simulink model "ROPOD_4Wheel_TdistZMPC_cntr_EC"  (R2017b)
settings: Solver=ode1  StartTime=0.0  StopTime=Tfinal  FixedStep=Ts  RelTol=1e-3  EnableMultiTasking=on
PreLoadFcn:
  | init_model
InitFcn:
  | init_model
values from neighbouring files (symbols this model uses):
  b_cx = 70.26    [RoPod_parameters.mat]
  b_cy = 36.5    [RoPod_parameters.mat]
  FFtheta_intia = 0    [init_model.m]
  FFxy_mass = 80    [init_model.m]
  I_fhz_dtheta_cntr = 0.5    [init_model.m]
  I_fhz_dvarphi_cntr = 0    [init_model.m]
  I_fhz_dxdy_cntr = 0.25    [init_model.m]
  k_cx = 4300    [RoPod_parameters.mat]
  k_cy = 4489    [RoPod_parameters.mat]
  K_gain_dtheta_cntr = 150    [init_model.m]
  K_gain_dvarphi_cntr = 0.05    [init_model.m]
  K_gain_dxdy_cntr = 200    [init_model.m]
  LL_wp_fhz_dtheta_cntr = 20    [init_model.m]
  LL_wp_fhz_dvarphi_cntr = 20    [init_model.m]
  LL_wp_fhz_dxdy_cntr = 20    [init_model.m]
  LL_wz_fhz_dtheta_cntr = 20    [init_model.m]
  LL_wz_fhz_dvarphi_cntr = 2    [init_model.m]
  LL_wz_fhz_dxdy_cntr = 20    [init_model.m]
  LPF_fhz_dtheta_cntr = 100    [init_model.m]
  LPF_fhz_dvarphi_cntr = 100    [init_model.m]
  LPF_fhz_dxdy_cntr = 100    [init_model.m]
  max_hw_tau = 7.0    (= 7)    [init_model.m]
  max_ropod_acc_theta = 1.6    [init_model.m]
  max_ropod_acc_xy = 1.0    (= 1)    [init_model.m]
  max_ropod_vel_theta = 1.6    [init_model.m]
  max_ropod_vel_xy = 1.0    (= 1)    [init_model.m]
  max_sw_current = 10    [init_model.m]
  Nwheels = 4    [init_model.m]
  pivot_offs_sws = [2.21 1.873 2.001 3.508]    [init_model.m]
  SW_COM1_ENABLE1 = hex2dec('0001')    [init_model.m]
  SW_COM1_ENABLE2 = hex2dec('0002')    [init_model.m]
  SW_COM1_MODE_TORQUE = bitshift(hex2dec('0000'),2)    [init_model.m]
  SW_COM1_MODE_VELOCITY = bitshift(hex2dec('0002'),2)    [init_model.m]
  SW_COM1_USE_TS = hex2dec('8000')    [init_model.m]
  sw_tau_2_curr = 1/motor_physical_parameters.torqueconstant.value    [init_model.m]
  Taucompfactor = 2.0    (= 2)    [init_model.m]
  Tinit = 1*Tslot    [init_model.m]
  Ts = 0.001    [init_model.m]
  Ts_MPC = 0.001    [init_model.m]
  xA = [1 -1 0 0 0 0 0.0206696424966 -0.0206696424966 0 0 0.0298227588181 -0.0298227588181 ... (4080 elements, 102x40)]    [ZMPCx_parameters.mat]
  xBd_dis = [1.12932348493e-06 0.000225071897401 0 0]    [ZMPCx_parameters.mat]
  xF = [0 0 0 0 0 0 0 0 0 0 0 0 ... (80 elements, 20x4)]    [ZMPCx_parameters.mat]
  xH = [20 0 0 0 0 0 0 0 0 0 0 0 ... (1600 elements, 40x40)]    [ZMPCx_parameters.mat]
  xPhi = [0.995143909015 -0.967809158823 0 0 0.980727027327 -1.91066813489 0 0 0.957042868744 -2.81984596436 0 0 ... (320 elements, 80x4)]    [ZMPCx_parameters.mat]
  xrho = 144000    [ZMPCx_parameters.mat]
  xW = [0 0 -4300 4300 0 0 -4211.12053726 4211.12053726 0 0 -4082.88267435 4082.88267435 ... (328 elements, 82x4)]    [ZMPCx_parameters.mat]
  yA = [1 -1 0 0 0 0 0.0146537039222 -0.0146537039222 0 0 0.0255124036215 -0.0255124036215 ... (4080 elements, 102x40)]    [ZMPCy_parameters.mat]
  yBd_dis = [1.24492522358e-06 0.000248362591603 0 0]    [ZMPCy_parameters.mat]
  yF = [0.00191047141222 0.00156448969707 0.00119761396088 0.000813779538874 0.00041715000072 1.20724055612e-05 -0.00039696993291 -0.000805406662726 -0.00120863105559 -0.00160205155743 -0.00198114365531 -0.00234150147928 ... (80 elements, 20x4)]    [ZMPCy_parameters.mat]
  yH = [2.00000002801 0 2.31602594113e-08 0 1.80085634996e-08 0 1.26053094289e-08 0 7.00898668547e-09 0 1.2808124932e-09 0 ... (1600 elements, 40x40)]    [ZMPCy_parameters.mat]
  yPhi = [0.994411530671 -1.11489967371 0 0 0.977778317439 -2.20691845877 0 0 0.950389393786 -3.2640842851 0 0 ... (320 elements, 80x4)]    [ZMPCy_parameters.mat]
  yrho = 10000    [ZMPCy_parameters.mat]
  yW = [0 0 -4489 4489 0 0 -4423.21952309 4423.21952309 0 0 -4308.69434324 4308.69434324 ... (328 elements, 82x4)]    [ZMPCy_parameters.mat]
undefined symbols (not defined in the file or in its folder): DiscIntNeverNeededParam, Fd_max, Fd_min, Fr_max, Fr_min, ropod_kinmodel_param
libraries: cstblocks x85, simulink x41, SOEM_EtherCAT_Lib x5
(part 1 of 5)
settings Model: SimulationMode=external  Creator=cesar  LastModifiedBy=root
settings OptimizationCC: PassReuseOutputArgsThreshold=0  MaxStackSize=64
settings DebuggingCC: ParameterTunabilityLossMsg=error
settings HardwareCC: ProdBitPerLong=64  ProdHWDeviceType=Intel->x86-64 (Linux 64)  TargetBitPerLong=64  TargetBitPerPointer=64  TargetBitPerSizeT=64  TargetBitPerPtrDiffT=64  TargetLargestAtomicFloat=Float  TargetIntDivRoundTo=Zero  TargetEndianess=LittleEndian  TargetWordSize=64  TargetHWDeviceType=Intel->x86-64 (Linux 64)
settings SFSimCC: MATLABDynamicMemAlloc=off
settings RTWCC: SystemTargetFile=mttarget.tlc  MakeCommand="make_rtw  CC=\"ccache gcc\" OPTS=\"-DNETIF_ID=0 -DTEST_CONN_MODEL -D_GNU_SOURCE -DPRIO=99\""  TemplateMakefile=mt_unix.tmf  Description=Generic Real-Time Target  CustomInclude=/usr/local/include/soem  Toolchain=Catkin  BuildConfiguration=Faster Runs  RTWCompilerOptimization=Custom  RTWCustomCompilerOptimizations=-O2 -g -W
settings RTWCC: CustomLibrary=|
  | /usr/local/lib/libsoem.so
  | libgamepad.so.1
settings CodeAppCC: ForceParamTrailComments=on  OperatorAnnotations=on
settings GRTTargetCC: TargetLangStandard=C89/C90 (ANSI)  UseToolchainInfoCompliant=off  ExtMode=on

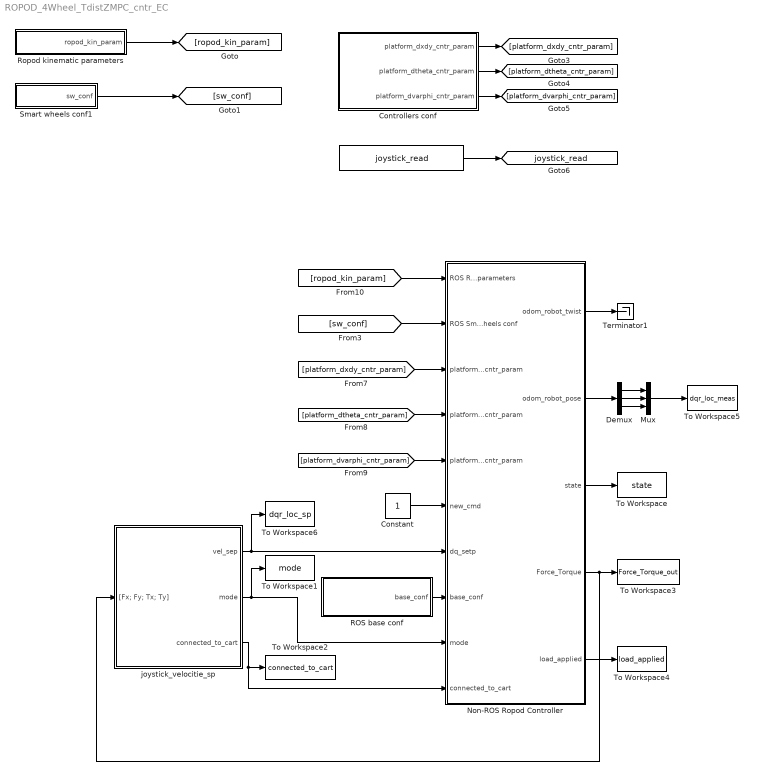
== system ROPOD_4Wheel_TdistZMPC_cntr_EC ==
  " " : S-Function  FunctionName=joystick_read  SFunctionDeploymentMode=off  EnableBusSupport=off  mask(Legacy Function){SFunctionSpec=double y1 = read_joystick(), ShowSpec=off}
      mask prompts: ShowSpec "Display function specification"
      mask help:
      | This block allows you to call the legacy functions specified by the following Legacy Code Tool definition:
      | def.SFunctionName = 'joystick_read';
      | def.OutputFcnSpec = 'double y1 = read_joystick()';
      | def.StartFcnSpec = 'void init()';
      | def.HeaderFiles = {'joystick.h', 'stdio.h', 'ncurses.h', 'gamepad.h'};
      | def.SourceFiles = {'joystick.c'};
      | def.HostLibFiles = {'libgamepad.so.1'};
      mask Help: <p>This block was generated automatically by the Legacy Code Tool. For detailed help on this tool, call<a href="matlab:legacy_code('help')"> legacy_code('help')</a>.</p>
      mask Callback ShowSpec:
      | if strcmp(get_param(gcbh, 'ShowSpec'), 'on')
      |   set_param(gcbh, 'MaskDisplay', sprintf('fprintf(''%s'');', get_param(gcbh, 'SFunctionSpec')));
      | else
      |   set_param(gcbh, 'MaskDisplay', sprintf('fprintf(''%s'');', get_param(gcbh, 'FunctionName')));
      | end
      mask Display: fprintf('joystick_read');
  Constant : Constant
  Controllers conf : Subsystem
  Demux : Demux  Outputs=3
  Mux : Mux  Inputs=3
  Non-ROS Ropod Controller : Subsystem
  ROS base conf : Subsystem
  Ropod kinematic parameters : Subsystem
  Smart wheels conf1 : Subsystem
  Terminator1 : Terminator
  To Workspace : ToWorkspace  VariableName=state  SampleTime=-1
      settings: Save2DSignal=2-D array (concatenate along first dimension)
  To Workspace1 : ToWorkspace  VariableName=mode  SampleTime=-1
      settings: Save2DSignal=2-D array (concatenate along first dimension)
  To Workspace2 : ToWorkspace  VariableName=connected_to_cart  SampleTime=-1
      settings: Save2DSignal=2-D array (concatenate along first dimension)
  To Workspace3 : ToWorkspace  VariableName=Force_Torque_out  SampleTime=-1
      settings: Save2DSignal=2-D array (concatenate along first dimension)
  To Workspace4 : ToWorkspace  VariableName=load_applied  SampleTime=-1
      settings: Save2DSignal=2-D array (concatenate along first dimension)
  To Workspace5 : ToWorkspace  VariableName=dqr_loc_meas  SampleTime=-1
      settings: Save2DSignal=2-D array (concatenate along first dimension)
  To Workspace6 : ToWorkspace  VariableName=dqr_loc_sp  SampleTime=-1
      settings: Save2DSignal=2-D array (concatenate along first dimension)
  joystick_velocitie_sp : Subsystem
  tag scope: joystick_read=global
  wires:
  Mux/1 -> To Workspace5/1
  Constant/1 -> Non-ROS Ropod Controller/6(new_cmd)
  " "/1 -> [joystick_read]
  [platform_dtheta_cntr_param] -> Non-ROS Ropod Controller/4(platform_dtheta_cntr_param)
  Non-ROS Ropod Controller/2(odom_robot_pose) -> Demux/1
  Demux/2 -> Mux/2
  [platform_dxdy_cntr_param] -> Non-ROS Ropod Controller/3(platform_dxdy_cntr_param)
  [platform_dvarphi_cntr_param] -> Non-ROS Ropod Controller/5(platform_dvarphi_cntr_param)
  Controllers conf/3(platform_dvarphi_cntr_param) -> [platform_dvarphi_cntr_param]
  Demux/3 -> Mux/3
  [ropod_kin_param] -> Non-ROS Ropod Controller/1(ROS Ropod kinematic parameters)
  Controllers conf/1(platform_dxdy_cntr_param) -> [platform_dxdy_cntr_param]
  Controllers conf/2(platform_dtheta_cntr_param) -> [platform_dtheta_cntr_param]
  [sw_conf] -> Non-ROS Ropod Controller/2(ROS Smart wheels conf)
  Ropod kinematic parameters/1(ropod_kin_param) -> [ropod_kin_param]
  Smart wheels conf1/1(sw_conf) -> [sw_conf]
  Non-ROS Ropod Controller/1(odom_robot_twist) -> Terminator1/1
  Demux/1 -> Mux/1
  ROS base conf/1(base_conf) -> Non-ROS Ropod Controller/8(base_conf)
  joystick_velocitie_sp/1(vel_sep) -> Non-ROS Ropod Controller/7(dq_setp), To Workspace6/1
  joystick_velocitie_sp/2(mode) -> Non-ROS Ropod Controller/9(mode), To Workspace1/1
  joystick_velocitie_sp/3(connected_to_cart) -> To Workspace2/1, Non-ROS Ropod Controller/10(connected_to_cart)
  Non-ROS Ropod Controller/3(state) -> To Workspace/1
  Non-ROS Ropod Controller/4(Force_Torque) -> joystick_velocitie_sp/1("[Fx; Fy; Tx; Ty]"), To Workspace3/1
  Non-ROS Ropod Controller/5(load_applied) -> To Workspace4/1

== system ROPOD_4Wheel_TdistZMPC_cntr_EC/Controllers conf ==
  Bus Creator : BusCreator  Inputs=5
  Bus Creator1 : BusCreator  Inputs=5
  Bus Creator2 : BusCreator  Inputs=5
  Constant1 : Constant  Value=I_fhz_dxdy_cntr
  Constant10 : Constant  Value=K_gain_dtheta_cntr
  Constant11 : Constant  Value=K_gain_dvarphi_cntr
  Constant12 : Constant  Value=I_fhz_dvarphi_cntr
  Constant13 : Constant  Value=LL_wp_fhz_dvarphi_cntr
  Constant14 : Constant  Value=LL_wz_fhz_dvarphi_cntr
  Constant15 : Constant  Value=LPF_fhz_dvarphi_cntr
  Constant2 : Constant  Value=LL_wp_fhz_dxdy_cntr
  Constant3 : Constant  Value=LL_wz_fhz_dxdy_cntr
  Constant4 : Constant  Value=LPF_fhz_dxdy_cntr
  Constant5 : Constant  Value=I_fhz_dtheta_cntr
  Constant6 : Constant  Value=LL_wp_fhz_dtheta_cntr
  Constant7 : Constant  Value=K_gain_dxdy_cntr
  Constant8 : Constant  Value=LL_wz_fhz_dtheta_cntr
  Constant9 : Constant  Value=LPF_fhz_dtheta_cntr
  platform_dxdy_cntr_param : Outport
  platform_dtheta_cntr_param : Outport  Port=2
  platform_dvarphi_cntr_param : Outport  Port=3
  wires:
  Constant2/1 -> Bus Creator/4  "LL_pole_fhz"
  Constant4/1 -> Bus Creator/5  "LPF_fhz"
  Bus Creator/1 -> platform_dxdy_cntr_param/1
  Constant1/1 -> Bus Creator/2  "I_freq_hz"
  Constant3/1 -> Bus Creator/3  "LL_zero_fhz"
  Constant7/1 -> Bus Creator/1  "P_gain"
  Bus Creator1/1 -> platform_dtheta_cntr_param/1
  Bus Creator2/1 -> platform_dvarphi_cntr_param/1
  Constant5/1 -> Bus Creator1/2  "I_freq_hz"
  Constant6/1 -> Bus Creator1/4  "LL_pole_fhz"
  Constant10/1 -> Bus Creator1/1  "P_gain"
  Constant8/1 -> Bus Creator1/3  "LL_zero_fhz"
  Constant9/1 -> Bus Creator1/5  "LPF_fhz"
  Constant15/1 -> Bus Creator2/5  "LPF_fhz"
  Constant12/1 -> Bus Creator2/2  "I_freq_hz"
  Constant14/1 -> Bus Creator2/3  "LL_zero_fhz"
  Constant11/1 -> Bus Creator2/1  "P_gain"
  Constant13/1 -> Bus Creator2/4  "LL_pole_fhz"

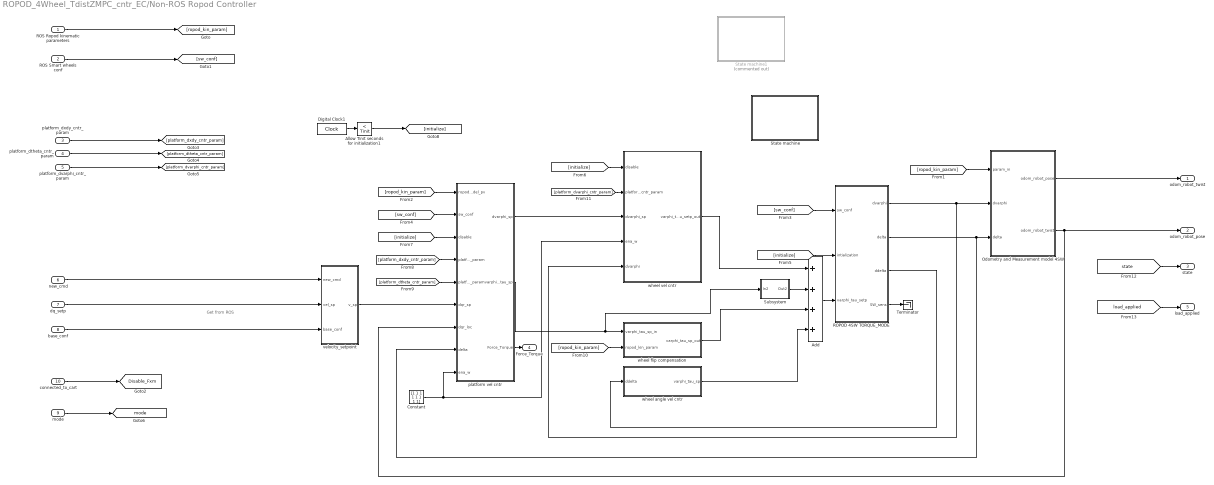
== system ROPOD_4Wheel_TdistZMPC_cntr_EC/Non-ROS Ropod Controller ==
  note: Get from ROS
  ROS Ropod kinematic parameters : Inport
  ROS Smart wheels conf : Inport  Port=2
  platform_dxdy_cntr_param : Inport  Port=3
  platform_dtheta_cntr_param : Inport  Port=4
  platform_dvarphi_cntr_param : Inport  Port=5
  new_cmd : Inport  Port=6
  dq_setp : Inport  Port=7
  base_conf : Inport  Port=8
  mode : Inport  Port=9
  connected_to_cart : Inport  Port=10
  Add : Sum  Inputs=++++
  Allow Tinit seconds for initialization1 : simulink/Logic and Bit Operations/Compare To Constant  relop=<  const=Tinit  OutDataTypeStr=boolean
  Constant : Constant  Value=[1 1 1 1 1 1 1 1]
  Digital Clock1 : DigitalClock  SampleTime=Ts
  Odometry and Measurement model 4SW : Subsystem
  ROPOD 4SW TORQUE_MODE : Subsystem
  State machine : Subsystem
  State machine1 : Subsystem  Commented=on
  Subsystem : Subsystem
  Terminator : Terminator
  platform vel cntr : Subsystem
  velocity_setpoint : Subsystem
  wheel angle vel cntr : Subsystem
  wheel flip compensation : Subsystem
  wheel vel cntr : Subsystem
  odom_robot_twist : Outport
  odom_robot_pose : Outport  Port=2
  state : Outport  Port=3
  Force_Torque : Outport  Port=4
  load_applied : Outport  Port=5
  tag scope: Disable_Fxm=global, mode=global
  wires:
  [sw_conf] -> ROPOD 4SW TORQUE_MODE/1(sw_conf)
  ROPOD 4SW TORQUE_MODE/3(ddelta) -> wheel angle vel cntr/1(ddelta)
  [initialize] -> wheel vel cntr/1(disable)
  base_conf/1 -> velocity_setpoint/3(base_conf)
  Digital Clock1/1 -> Allow Tinit seconds for initialization1/1
  [sw_conf] -> platform vel cntr/2(sw_conf)
  [platform_dvarphi_cntr_param] -> wheel vel cntr/2(platform_dxdy_cntr_param)
  wheel angle vel cntr/1(varphi_tau_sp) -> Add/4
  ROPOD 4SW TORQUE_MODE/2(delta) -> Odometry and Measurement model 4SW/3(delta), platform vel cntr/8(delta)
  [platform_dtheta_cntr_param] -> platform vel cntr/5(platform_dtheta_cntr_param)
  platform vel cntr/2(varphi_tau_sp) -> Subsystem/1(In2), wheel flip compensation/1(varphi_tau_sp_in)
  Add/1 -> ROPOD 4SW TORQUE_MODE/3(varphi_tau_setp)
  [platform_dxdy_cntr_param] -> platform vel cntr/4(platform_dxdy_cntr_param)
  [ropod_kin_param] -> platform vel cntr/1(ropod_kinmodel_pv)
  velocity_setpoint/1(v_sp) -> platform vel cntr/6(dqr_sp)
  wheel flip compensation/1(varphi_tau_sp_out) -> Add/3
  ROS Smart wheels conf/1 -> [sw_conf]
  platform_dvarphi_cntr_param/1 -> [platform_dvarphi_cntr_param]
  Odometry and Measurement model 4SW/1(odom_robot_pose) -> odom_robot_twist/1
  [ropod_kin_param] -> Odometry and Measurement model 4SW/1(param_in)
  [initialize] -> platform vel cntr/3(disable)
  ROPOD 4SW TORQUE_MODE/4(SW_sens) -> Terminator/1
  platform_dxdy_cntr_param/1 -> [platform_dxdy_cntr_param]
  ROS Ropod kinematic parameters/1 -> [ropod_kin_param]
  [initialize] -> ROPOD 4SW TORQUE_MODE/2(intialization)
  [ropod_kin_param] -> wheel flip compensation/2(ropod_kin_param)
  platform vel cntr/1(dvarphi_sp) -> wheel vel cntr/3(dvarphi_sp)
  Odometry and Measurement model 4SW/2(odom_robot_twist) -> odom_robot_pose/1, platform vel cntr/7(dqr_loc)
  ROPOD 4SW TORQUE_MODE/1(dvarphi) -> Odometry and Measurement model 4SW/2(dvarphi), wheel vel cntr/5(dvarphi)
  platform_dtheta_cntr_param/1 -> [platform_dtheta_cntr_param]
  new_cmd/1 -> velocity_setpoint/1(new_cmd)
  dq_setp/1 -> velocity_setpoint/2(vel_sp)
  Constant/1 -> wheel vel cntr/4(ena_w), platform vel cntr/9(ena_w)
  Allow Tinit seconds for initialization1/1 -> [initialize]
  wheel vel cntr/1(varphi_tau_setp_out) -> Add/1
  Subsystem/1(Out2) -> Add/2
  connected_to_cart/1 -> [Disable_Fxm]
  mode/1 -> [mode]
  [state] -> state/1
  platform vel cntr/3(Force_Torque) -> Force_Torque/1
  [load_applied] -> load_applied/1

== system ROPOD_4Wheel_TdistZMPC_cntr_EC/ROS base conf ==
  Bus Creator : BusCreator  Inputs=4
  Constant : Constant  Value=max_ropod_vel_xy  SampleTime=Ts
  Constant1 : Constant  Value=max_ropod_acc_xy  SampleTime=Ts
  Constant2 : Constant  Value=max_ropod_vel_theta  SampleTime=Ts
  Constant3 : Constant  Value=max_ropod_acc_theta  SampleTime=Ts
  base_conf : Outport
  wires:
  Constant1/1 -> Bus Creator/2  "max_acc_xy"
  Constant/1 -> Bus Creator/1  "max_vel_xy"
  Bus Creator/1 -> base_conf/1
  Constant3/1 -> Bus Creator/4  "max_acc_theta"
  Constant2/1 -> Bus Creator/3  "max_vel_theta"

== system ROPOD_4Wheel_TdistZMPC_cntr_EC/Ropod kinematic parameters ==
  Constant : Constant  Value=ropod_kinmodel_param.r_w(1)
  Constant1 : Constant  Value=ropod_kinmodel_param.r_w(2)
  Constant10 : Constant  Value=ropod_kinmodel_param.C_SW(1)
  Constant11 : Constant  Value=ropod_kinmodel_param.C_SW(2)
  Constant12 : Constant  Value=ropod_kinmodel_param.C_SW(3)
  Constant13 : Constant  Value=ropod_kinmodel_param.C_SW(4)
  Constant14 : Constant  Value=ropod_kinmodel_param.C_SW(5)
  Constant15 : Constant  Value=ropod_kinmodel_param.C_SW(6)
  Constant16 : Constant  Value=ropod_kinmodel_param.C_SW(7)
  Constant17 : Constant  Value=ropod_kinmodel_param.C_SW(8)
  Constant2 : Constant  Value=ropod_kinmodel_param.r_w(3)
  Constant3 : Constant  Value=ropod_kinmodel_param.r_w(4)
  Constant4 : Constant  Value=ropod_kinmodel_param.r_w(5)
  Constant5 : Constant  Value=ropod_kinmodel_param.r_w(6)
  Constant6 : Constant  Value=ropod_kinmodel_param.r_w(7)
  Constant7 : Constant  Value=ropod_kinmodel_param.r_w(8)
  Constant8 : Constant  Value=ropod_kinmodel_param.s_w
  Constant9 : Constant  Value=ropod_kinmodel_param.d_w
  Mux : Mux  Inputs=18
  ropod_kin_param : Outport
  wires:
  Mux/1 -> ropod_kin_param/1
  Constant3/1 -> Mux/4
  Constant6/1 -> Mux/7
  Constant5/1 -> Mux/6
  Constant1/1 -> Mux/2
  Constant2/1 -> Mux/3
  Constant/1 -> Mux/1
  Constant7/1 -> Mux/8
  Constant4/1 -> Mux/5
  Constant9/1 -> Mux/10
  Constant8/1 -> Mux/9
  Constant13/1 -> Mux/14
  Constant10/1 -> Mux/11
  Constant12/1 -> Mux/13
  Constant11/1 -> Mux/12
  Constant17/1 -> Mux/18
  Constant14/1 -> Mux/15
  Constant15/1 -> Mux/16
  Constant16/1 -> Mux/17

== system ROPOD_4Wheel_TdistZMPC_cntr_EC/Smart wheels conf1 ==
  Bus Creator : BusCreator  Inputs=6
  enable : Constant
  max_current : Constant  Value=max_sw_current
  pivot_offset_sw1 : Constant  Value=pivot_offs_sws(1)
  pivot_offset_sw2 : Constant  Value=pivot_offs_sws(2)
  pivot_offset_sw3 : Constant  Value=pivot_offs_sws(3)
  pivot_offset_sw4 : Constant  Value=pivot_offs_sws(4)
  sw_conf : Outport
  wires:
  enable/1 -> Bus Creator/1  "enable"
  Bus Creator/1 -> sw_conf/1
  max_current/1 -> Bus Creator/2  "max_current"
  pivot_offset_sw1/1 -> Bus Creator/3  "pivot_offs_sw1"
  pivot_offset_sw2/1 -> Bus Creator/4  "pivot_offs_sw2"
  pivot_offset_sw3/1 -> Bus Creator/5  "pivot_offs_sw3"
  pivot_offset_sw4/1 -> Bus Creator/6  "pivot_offs_sw4"

== system ROPOD_4Wheel_TdistZMPC_cntr_EC/joystick_velocitie_sp ==
  "[Fx; Fy; Tx; Ty]" : Inport
  Chart : Stateflow chart  TreatAsAtomicUnit=on
  vel_sep : Outport
  mode : Outport  Port=2
  connected_to_cart : Outport  Port=3
  wires:
  [joystick_read] -> Chart/1(joystick)
  Chart/1(velocity_sp) -> vel_sep/1
  [dqr_loc] -> Chart/2(robot_speed)
  Chart/2(mode) -> mode/1
  Chart/3(connected_to_cart) -> connected_to_cart/1
  "[Fx; Fy; Tx; Ty]"/1 -> Chart/3(Fx_Fy_Tx_Ty)

== system ROPOD_4Wheel_TdistZMPC_cntr_EC/Non-ROS Ropod Controller/Odometry and Measurement model 4SW ==
  note: This output is only useful when using ros
      | This data is fed to /odom/pose
  note: This part is in global coordinates
  note: This part is in local coordinates
  param_in : Inport
  dvarphi : Inport  Port=2
  delta : Inport  Port=3
  Discrete-Time Integrator : DiscreteIntegrator  InitialConditionSetting=State (most efficient)  SampleTime=Ts  ICPrevOutput=DiscIntNeverNeededParam  ICPrevScaledInput=DiscIntNeverNeededParam
  Jqwl_matrix : MATLAB Function  TreatAsAtomicUnit=on
  Product3 : Product  Multiplication=Matrix(*)
  Selector3 : Selector  InputPortWidth=3  IndexOptions=Index vector (dialog)  Indices=3  OutputSizes=1
  Signal Specification : SignalSpecification  Dimensions=[3 1]
  pos_rot_matrix : MATLAB Function  TreatAsAtomicUnit=on
  odom_robot_pose : Outport
  odom_robot_twist : Outport  Port=2
  wires:
  Product3/1 -> Signal Specification/1
  param_in/1 -> Jqwl_matrix/1(ropod_kinmodel_param_vec)
  delta/1 -> Jqwl_matrix/2(delta)
  Jqwl_matrix/1(Jqwl) -> Product3/1
  dvarphi/1 -> Product3/2
  Signal Specification/1 -> pos_rot_matrix/1(dqr_loc), odom_robot_twist/1
  Selector3/1 -> pos_rot_matrix/2(theta_odom)
  pos_rot_matrix/1(dqr_glb) -> Discrete-Time Integrator/1
  Discrete-Time Integrator/1 -> odom_robot_pose/1, Selector3/1

== system ROPOD_4Wheel_TdistZMPC_cntr_EC/Non-ROS Ropod Controller/ROPOD 4SW TORQUE_MODE ==
  sw_conf : Inport
  intialization : Inport  Port=2
  varphi_tau_setp : Inport  Port=3
  Bus Creator : BusCreator  Inputs=4
  Display1 : Display  Commented=on
  ECAT_Interface : SOEM_EtherCAT_Lib/ECAT_Interface  Priority=0  Commented=on  IFINTERFACE=eth0  TS=Ts
      settings: SourceProductName=SOEM_EtherCAT_Lib
  Gain1 : Gain  Commented=on  OutDataTypeStr=double
  Initialization switch : Subsystem
  ROPOD_4Wheel_sens : Subsystem
  ROPOD_4Wheel_torque_cmd : Subsystem
  Smart_Wheel_1 : Subsystem
  Smart_Wheel_2 : Subsystem
  Smart_Wheel_3 : Subsystem
  Smart_Wheel_4 : Subsystem
  Subsystem : Subsystem
  empywheel : Subsystem  Commented=on
  dvarphi : Outport
  delta : Outport  Port=2
  ddelta : Outport  Port=3
  SW_sens : Outport  Port=4
  wires:
  ROPOD_4Wheel_sens/2(delta) -> delta/1
  ROPOD_4Wheel_sens/1(dvarphi) -> dvarphi/1
  ECAT_Interface/1 -> Gain1/1
  Gain1/1 -> Display1/1
  ROPOD_4Wheel_sens/3(ddelta) -> ddelta/1
  ROPOD_4Wheel_torque_cmd/4(SW4_cmd) -> Smart_Wheel_4/1(SW4_cmd)
  ROPOD_4Wheel_torque_cmd/1(SW1_cmd) -> Smart_Wheel_1/1(SW1_cmd)
  ROPOD_4Wheel_torque_cmd/3(SW3_cmd) -> Smart_Wheel_3/1(SW3_cmd)
  sw_conf/1 -> ROPOD_4Wheel_torque_cmd/1(sw_conf), ROPOD_4Wheel_sens/2(sw_conf)
  ROPOD_4Wheel_torque_cmd/2(SW2_cmd) -> Smart_Wheel_2/1(SW2_cmd)
  Smart_Wheel_1/1(SW1_sens) -> Bus Creator/1, ROPOD_4Wheel_sens/3(SW1_sens)  "SW1_sens"
  Smart_Wheel_4/1(SW4_sens) -> ROPOD_4Wheel_sens/6(SW4_sens), Bus Creator/4  "SW4_sens"
  Smart_Wheel_2/1(SW2_sens) -> ROPOD_4Wheel_sens/4(SW2_sens), Bus Creator/2  "SW2_sens"
  Smart_Wheel_3/1(SW3_sens) -> ROPOD_4Wheel_sens/5(SW3_sens), Bus Creator/3  "SW3_sens"
  Bus Creator/1 -> SW_sens/1
  Initialization switch/1(cntr_mode) -> ROPOD_4Wheel_torque_cmd/2(cntr_mode)
  Initialization switch/2(wheel_setp) -> ROPOD_4Wheel_torque_cmd/3(wheel_setp)
  Subsystem/1(varphi_curr_setp) -> Initialization switch/2(In2)
  varphi_tau_setp/1 -> Subsystem/1(varphi_tau_setp)
  intialization/1 -> ROPOD_4Wheel_sens/1(disable), Initialization switch/1(vel_mode_enable)

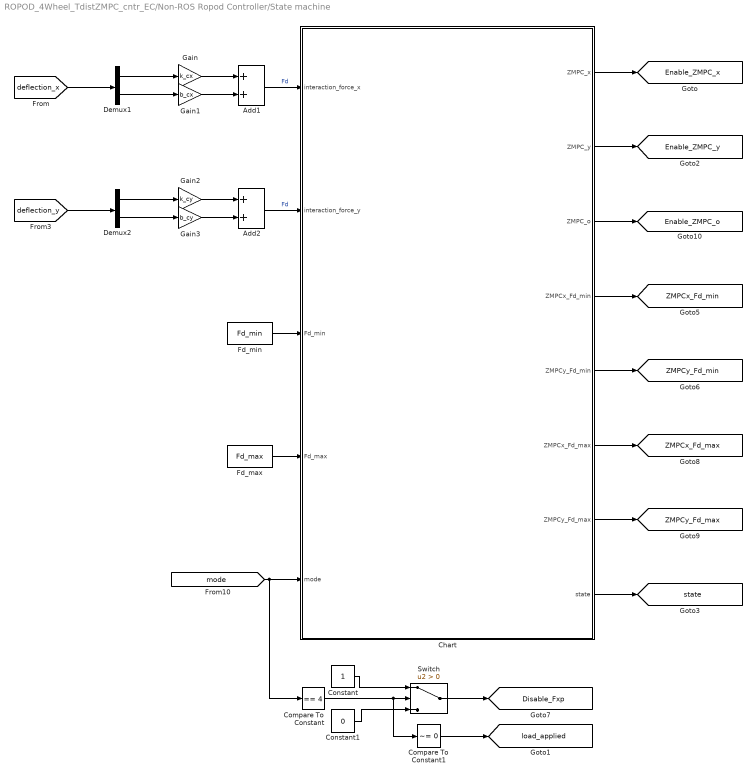
== system ROPOD_4Wheel_TdistZMPC_cntr_EC/Non-ROS Ropod Controller/State machine ==
  Add1 : Sum
  Add2 : Sum
  Chart : Stateflow chart  TreatAsAtomicUnit=on
  Compare To Constant : simulink/Logic and Bit Operations/Compare To Constant  relop===  const=4  OutDataTypeStr=boolean
  Compare To Constant1 : simulink/Logic and Bit Operations/Compare To Constant  relop=~=  const=0  OutDataTypeStr=boolean
  Constant : Constant
  Constant1 : Constant  Value=0
  Demux1 : Demux  Outputs=2
  Demux2 : Demux  Outputs=2
  Fd_max : Constant  Value=Fd_max
  Fd_min : Constant  Value=Fd_min
  Gain : Gain  Gain=k_cx
  Gain1 : Gain  Gain=b_cx
  Gain2 : Gain  Gain=k_cy
  Gain3 : Gain  Gain=b_cy
  Switch : Switch  Criteria=u2 > Threshold
  tag scope: Disable_Fxp=global, Enable_ZMPC_o=global, Enable_ZMPC_x=global, Enable_ZMPC_y=global, ZMPCx_Fd_max=global, ZMPCx_Fd_min=global, ZMPCy_Fd_max=global, ZMPCy_Fd_min=global, load_applied=global, state=global
  wires:
  Chart/2(ZMPC_y) -> [Enable_ZMPC_y]
  Demux1/1 -> Gain/1
  [deflection_y] -> Demux2/1
  Gain/1 -> Add1/1
  Add1/1 -> Chart/1(interaction_force_x)  "Fd"
  Add2/1 -> Chart/2(interaction_force_y)  "Fd"
  Fd_min/1 -> Chart/3(Fd_min)
  Demux2/1 -> Gain2/1
  [deflection_x] -> Demux1/1
  Gain3/1 -> Add2/2
  Demux2/2 -> Gain3/1
  Chart/1(ZMPC_x) -> [Enable_ZMPC_x]
  Gain1/1 -> Add1/2
  Demux1/2 -> Gain1/1
  Gain2/1 -> Add2/1
  [mode] -> Compare To Constant/1, Chart/5(mode)
  Chart/4(ZMPCx_Fd_min) -> [ZMPCx_Fd_min]
  Chart/5(ZMPCy_Fd_min) -> [ZMPCy_Fd_min]
  Fd_max/1 -> Chart/4(Fd_max)
  Chart/7(ZMPCy_Fd_max) -> [ZMPCy_Fd_max]
  Chart/6(ZMPCx_Fd_max) -> [ZMPCx_Fd_max]
  Chart/3(ZMPC_o) -> [Enable_ZMPC_o]
  Chart/8(state) -> [state]
  Compare To Constant/1 -> Compare To Constant1/1, Switch/2
  Constant1/1 -> Switch/3
  Constant/1 -> Switch/1
  Switch/1 -> [Disable_Fxp]
  Compare To Constant1/1 -> [load_applied]

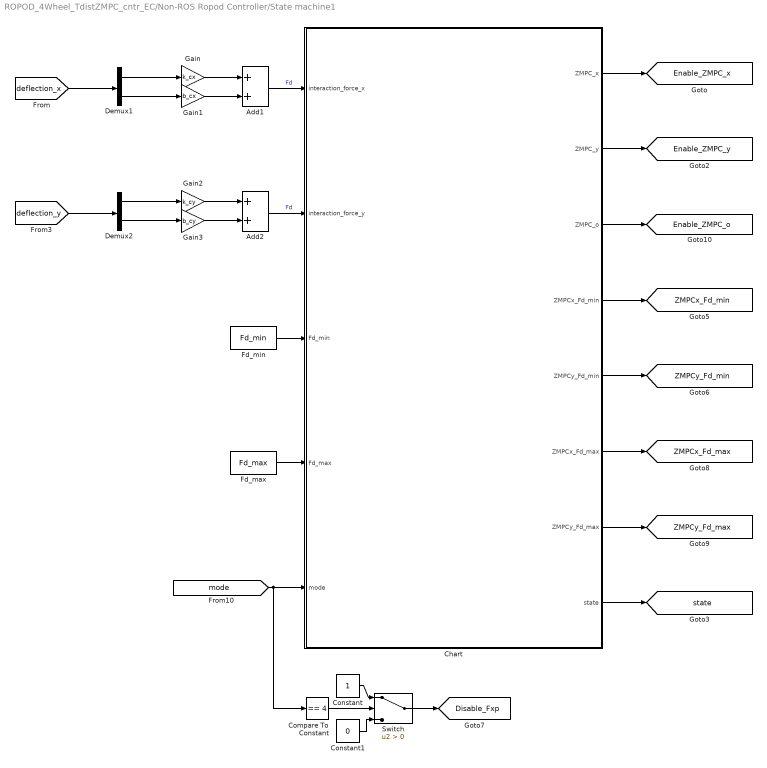
== system ROPOD_4Wheel_TdistZMPC_cntr_EC/Non-ROS Ropod Controller/State machine1 ==
  Add1 : Sum
  Add2 : Sum
  Chart : Stateflow chart  TreatAsAtomicUnit=on
  Compare To Constant : simulink/Logic and Bit Operations/Compare To Constant  relop===  const=4  OutDataTypeStr=boolean
  Constant : Constant
  Constant1 : Constant  Value=0
  Demux1 : Demux  Outputs=2
  Demux2 : Demux  Outputs=2
  Fd_max : Constant  Value=Fd_max
  Fd_min : Constant  Value=Fd_min
  Gain : Gain  Gain=k_cx
  Gain1 : Gain  Gain=b_cx
  Gain2 : Gain  Gain=k_cy
  Gain3 : Gain  Gain=b_cy
  Switch : Switch  Criteria=u2 > Threshold
  tag scope: Disable_Fxp=global, Enable_ZMPC_o=global, Enable_ZMPC_x=global, Enable_ZMPC_y=global, ZMPCx_Fd_max=global, ZMPCx_Fd_min=global, ZMPCy_Fd_max=global, ZMPCy_Fd_min=global, state=global
  wires:
  Chart/2(ZMPC_y) -> [Enable_ZMPC_y]
  Demux1/1 -> Gain/1
  [deflection_y] -> Demux2/1
  Gain/1 -> Add1/1
  Add1/1 -> Chart/1(interaction_force_x)  "Fd"
  Add2/1 -> Chart/2(interaction_force_y)  "Fd"
  Fd_min/1 -> Chart/3(Fd_min)
  Demux2/1 -> Gain2/1
  [deflection_x] -> Demux1/1
  Gain3/1 -> Add2/2
  Demux2/2 -> Gain3/1
  Chart/1(ZMPC_x) -> [Enable_ZMPC_x]
  Gain1/1 -> Add1/2
  Demux1/2 -> Gain1/1
  Gain2/1 -> Add2/1
  [mode] -> Compare To Constant/1, Chart/5(mode)
  Chart/4(ZMPCx_Fd_min) -> [ZMPCx_Fd_min]
  Chart/5(ZMPCy_Fd_min) -> [ZMPCy_Fd_min]
  Fd_max/1 -> Chart/4(Fd_max)
  Chart/7(ZMPCy_Fd_max) -> [ZMPCy_Fd_max]
  Chart/6(ZMPCx_Fd_max) -> [ZMPCx_Fd_max]
  Chart/3(ZMPC_o) -> [Enable_ZMPC_o]
  Chart/8(state) -> [state]
  Switch/1 -> [Disable_Fxp]
  Compare To Constant/1 -> Switch/2
  Constant1/1 -> Switch/3
  Constant/1 -> Switch/1

== system ROPOD_4Wheel_TdistZMPC_cntr_EC/Non-ROS Ropod Controller/Subsystem ==
  In2 : Inport
  Constant1 : Constant  Value=0
  Logical Operator : Logic  Operator=OR  Inputs=3  AllPortsSameDT=off  OutDataTypeStr=boolean
  Switch1 : Switch  Criteria=u2 > Threshold
  Out2 : Outport
  wires:
  [Enable_ZMPC_o] -> Logical Operator/3
  Constant1/1 -> Switch1/1
  Logical Operator/1 -> Switch1/2
  [Enable_ZMPC_x] -> Logical Operator/1
  Switch1/1 -> Out2/1
  In2/1 -> Switch1/3
  [Enable_ZMPC_y] -> Logical Operator/2

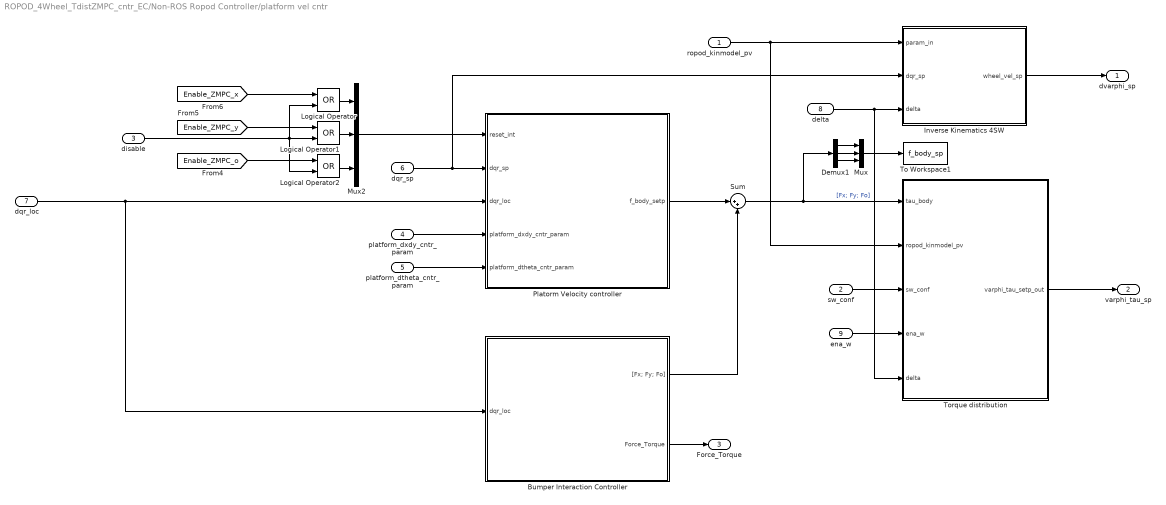
== system ROPOD_4Wheel_TdistZMPC_cntr_EC/Non-ROS Ropod Controller/platform vel cntr ==
  ropod_kinmodel_pv : Inport
  sw_conf : Inport  Port=2
  disable : Inport  Port=3
  platform_dxdy_cntr_param : Inport  Port=4
  platform_dtheta_cntr_param : Inport  Port=5
  dqr_sp : Inport  Port=6
  dqr_loc : Inport  Port=7
  delta : Inport  Port=8
  ena_w : Inport  Port=9
  Bumper Interaction Controller : Subsystem
  Demux1 : Demux  Outputs=3
  Inverse Kinematics 4SW : Subsystem
  Logical Operator : Logic  Operator=OR  AllPortsSameDT=off  OutDataTypeStr=boolean
  Logical Operator1 : Logic  Operator=OR  AllPortsSameDT=off  OutDataTypeStr=boolean
  Logical Operator2 : Logic  Operator=OR  AllPortsSameDT=off  OutDataTypeStr=boolean
  Mux : Mux  Inputs=3
  Mux2 : Mux  Inputs=3
  Platorm Velocity controller : Subsystem
  Sum : Sum  Inputs=|++
  To Workspace1 : ToWorkspace  VariableName=f_body_sp  SampleTime=-1
      settings: Save2DSignal=2-D array (concatenate along first dimension)
  Torque distribution : Subsystem
  dvarphi_sp : Outport
  varphi_tau_sp : Outport  Port=2
  Force_Torque : Outport  Port=3
  wires:
  delta/1 -> Torque distribution/5(delta), Inverse Kinematics 4SW/3(delta)
  ena_w/1 -> Torque distribution/4(ena_w)
  sw_conf/1 -> Torque distribution/3(sw_conf)
  Torque distribution/1(varphi_tau_setp_out) -> varphi_tau_sp/1
  ropod_kinmodel_pv/1 -> Inverse Kinematics 4SW/1(param_in), Torque distribution/2(ropod_kinmodel_pv)
  Inverse Kinematics 4SW/1(wheel_vel_sp) -> dvarphi_sp/1
  platform_dxdy_cntr_param/1 -> Platorm Velocity controller/4(platform_dxdy_cntr_param)
  platform_dtheta_cntr_param/1 -> Platorm Velocity controller/5(platform_dtheta_cntr_param)
  Platorm Velocity controller/1(f_body_setp) -> Sum/1
  dqr_sp/1 -> Inverse Kinematics 4SW/2(dqr_sp), Platorm Velocity controller/2(dqr_sp)
  dqr_loc/1 -> Bumper Interaction Controller/1(dqr_loc), Platorm Velocity controller/3(dqr_loc)
  Bumper Interaction Controller/1("[Fx; Fy; Fo]") -> Sum/2
  Mux2/1 -> Platorm Velocity controller/1(reset_int)
  Logical Operator/1 -> Mux2/1
  [Enable_ZMPC_x] -> Logical Operator/1
  Logical Operator1/1 -> Mux2/2
  [Enable_ZMPC_y] -> Logical Operator1/1
  Logical Operator2/1 -> Mux2/3
  disable/1 -> Logical Operator2/2, Logical Operator/2, Logical Operator1/2
  [Enable_ZMPC_o] -> Logical Operator2/1
  Bumper Interaction Controller/2(Force_Torque) -> Force_Torque/1
  Demux1/1 -> Mux/1
  Sum/1 -> Demux1/1, Torque distribution/1(tau_body)  "[Fx; Fy; Fo]"
  Mux/1 -> To Workspace1/1
  Demux1/2 -> Mux/2
  Demux1/3 -> Mux/3

== system ROPOD_4Wheel_TdistZMPC_cntr_EC/Non-ROS Ropod Controller/velocity_setpoint ==
  new_cmd : Inport
  vel_sp : Inport  Port=2
  base_conf : Inport  Port=3
  Acceleration and Velocity Limits : Subsystem
  Acceleration and Velocity Limits1 : Subsystem
  Constant1 : Constant  Value=0
  Constant2 : Constant  Value=0
  Constant3 : Constant  Value=0
  Demux1 : Demux  Outputs=3
  Mux : Mux  Inputs=3.
  Switch1 : Switch  Criteria=u2 > Threshold
  Switch2 : Switch  Criteria=u2 > Threshold
  Switch3 : Switch  Criteria=u2 > Threshold
  v_sp : Outport
  wires:
  Demux1/3 -> Switch3/3
  Demux1/1 -> Switch1/3
  Acceleration and Velocity Limits/1(dq_loc) -> v_sp/1
  Demux1/2 -> Switch2/3
  [Enable_ZMPC_x] -> Switch1/2
  [Enable_ZMPC_y] -> Switch2/2
  [Enable_ZMPC_o] -> Switch3/2
  Constant1/1 -> Switch1/1
  Constant2/1 -> Switch2/1
  Constant3/1 -> Switch3/1
  Switch1/1 -> Mux/1
  Switch2/1 -> Mux/2
  Switch3/1 -> Mux/3
  Mux/1 -> Acceleration and Velocity Limits/1(dq_setp)
  base_conf/1 -> Acceleration and Velocity Limits/2(base_conf)
  new_cmd/1 -> Acceleration and Velocity Limits1/1(new_cmd)
  vel_sp/1 -> Acceleration and Velocity Limits1/2(dq_setp)
  Acceleration and Velocity Limits1/1(dq_loc) -> Demux1/1

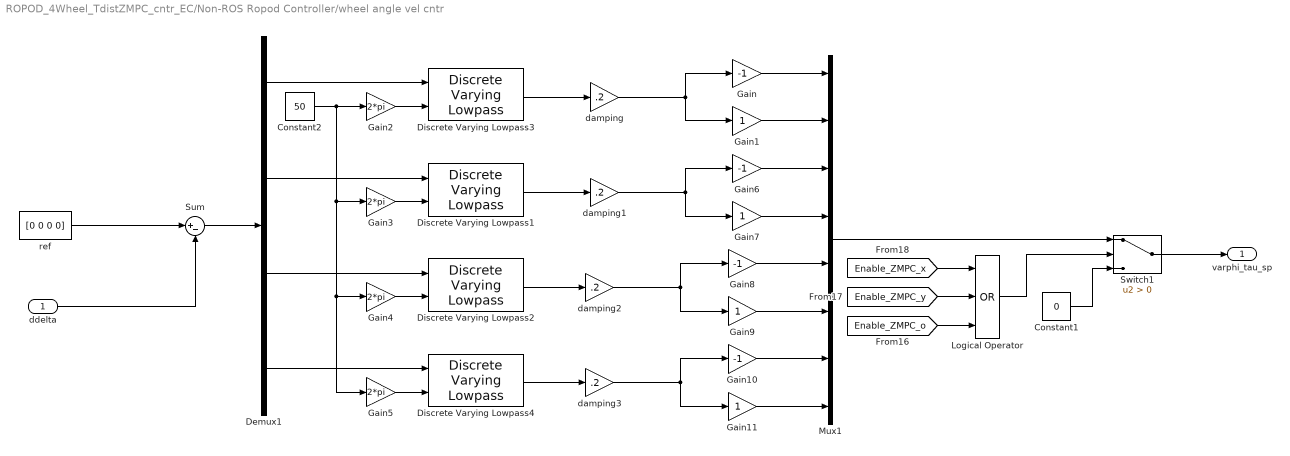
== system ROPOD_4Wheel_TdistZMPC_cntr_EC/Non-ROS Ropod Controller/wheel angle vel cntr ==
  ddelta : Inport
  Constant1 : Constant  Value=0
  Constant2 : Constant  Value=50
  Demux1 : Demux
  Discrete Varying Lowpass{1..4} (4 alike) : cstblocks/Linear Parameter Varying/Discrete Varying Lowpass  N=1  w0=0  Ts=Ts
      settings: SourceProductName=Control System Toolbox  SourceProductBaseCode=CT
  Gain{,6,8,10} (4 alike) : Gain  Gain=-1
  Gain{1,7,9,11} (4 alike) : Gain
  Gain{2..5} (4 alike) : Gain  Gain=2*pi
  Logical Operator : Logic  Operator=OR  Inputs=3  AllPortsSameDT=off  OutDataTypeStr=boolean
  Mux1 : Mux  Inputs=8
  Sum : Sum  Inputs=|+-
  Switch1 : Switch  Criteria=u2 > Threshold
  damping{,1..3} (4 alike) : Gain  Gain=.2
  ref : Constant  Value=[0 0 0 0]
  varphi_tau_sp : Outport
  wires:
  Demux1/2 -> Discrete Varying Lowpass1/1
  ddelta/1 -> Sum/2
  Demux1/3 -> Discrete Varying Lowpass2/1
  Demux1/4 -> Discrete Varying Lowpass4/1
  damping/1 -> Gain1/1, Gain/1
  Gain1/1 -> Mux1/2
  ref/1 -> Sum/1
  Sum/1 -> Demux1/1
  Gain/1 -> Mux1/1
  Gain2/1 -> Discrete Varying Lowpass3/2
  Gain3/1 -> Discrete Varying Lowpass1/2
  Gain4/1 -> Discrete Varying Lowpass2/2
  Constant2/1 -> Gain5/1, Gain4/1, Gain3/1, Gain2/1
  Gain5/1 -> Discrete Varying Lowpass4/2
  Demux1/1 -> Discrete Varying Lowpass3/1
  Discrete Varying Lowpass3/1 -> damping/1
  Discrete Varying Lowpass1/1 -> damping1/1
  damping1/1 -> Gain6/1, Gain7/1
  damping2/1 -> Gain9/1, Gain8/1
  Discrete Varying Lowpass2/1 -> damping2/1
  Discrete Varying Lowpass4/1 -> damping3/1
  damping3/1 -> Gain10/1, Gain11/1
  Gain11/1 -> Mux1/8
  Gain10/1 -> Mux1/7
  Gain9/1 -> Mux1/6
  Gain8/1 -> Mux1/5
  Gain7/1 -> Mux1/4
  Gain6/1 -> Mux1/3
  Logical Operator/1 -> Switch1/2
  Mux1/1 -> Switch1/1
  [Enable_ZMPC_o] -> Logical Operator/3
  [Enable_ZMPC_y] -> Logical Operator/2
  Switch1/1 -> varphi_tau_sp/1
  Constant1/1 -> Switch1/3
  [Enable_ZMPC_x] -> Logical Operator/1

== system ROPOD_4Wheel_TdistZMPC_cntr_EC/Non-ROS Ropod Controller/wheel flip compensation ==
  varphi_tau_sp_in : Inport
  ropod_kin_param : Inport  Port=2
  Constant : Constant  Value=3
  Constant1 : Constant  Value=0
  Demux : Demux  Outputs=8
  Logical Operator : Logic  Operator=OR  Inputs=3  AllPortsSameDT=off  OutDataTypeStr=boolean
  MATLAB Function : MATLAB Function  TreatAsAtomicUnit=on
  MATLAB Function1 : MATLAB Function  TreatAsAtomicUnit=on
  MATLAB Function2 : MATLAB Function  TreatAsAtomicUnit=on
  MATLAB Function3 : MATLAB Function  TreatAsAtomicUnit=on
  Mux : Mux  Inputs=8
  Switch1 : Switch  Criteria=u2 > Threshold
  Terminator : Terminator
  varphi_tau_sp_out : Outport
  wires:
  varphi_tau_sp_in/1 -> Demux/1
  ropod_kin_param/1 -> [ropod_kin_param]
  Constant/1 -> [kmax]
  Demux/2 -> MATLAB Function/2(tr)
  Demux/1 -> MATLAB Function/1(tl)
  [kmax] -> MATLAB Function/4(kmax)
  [ropod_kin_param] -> MATLAB Function/3(ropod_kinmodel_param_vec)
  Demux/4 -> MATLAB Function1/2(tr)
  Demux/3 -> MATLAB Function1/1(tl)
  [kmax] -> MATLAB Function1/4(kmax)
  [ropod_kin_param] -> MATLAB Function1/3(ropod_kinmodel_param_vec)
  Demux/6 -> MATLAB Function2/2(tr)
  Demux/5 -> MATLAB Function2/1(tl)
  [kmax] -> MATLAB Function2/4(kmax)
  [ropod_kin_param] -> MATLAB Function2/3(ropod_kinmodel_param_vec)
  Demux/8 -> MATLAB Function3/2(tr)
  Demux/7 -> MATLAB Function3/1(tl)
  [kmax] -> MATLAB Function3/4(kmax)
  [ropod_kin_param] -> MATLAB Function3/3(ropod_kinmodel_param_vec)
  MATLAB Function/1(tl_out) -> Mux/1
  MATLAB Function1/1(tl_out) -> Mux/3
  MATLAB Function2/1(tl_out) -> Mux/5
  MATLAB Function3/1(tl_out) -> Mux/7
  MATLAB Function/2(tr_out) -> Mux/2
  MATLAB Function1/2(tr_out) -> Mux/4
  MATLAB Function2/2(tr_out) -> Mux/6
  MATLAB Function3/2(tr_out) -> Mux/8
  MATLAB Function/3(sc) -> Terminator/1
  Logical Operator/1 -> Switch1/2
  Switch1/1 -> varphi_tau_sp_out/1
  [Enable_ZMPC_x] -> Logical Operator/1
  [Enable_ZMPC_y] -> Logical Operator/2
  [Enable_ZMPC_o] -> Logical Operator/3
  Constant1/1 -> Switch1/3
  Mux/1 -> Switch1/1

== system ROPOD_4Wheel_TdistZMPC_cntr_EC/Non-ROS Ropod Controller/wheel vel cntr ==
  disable : Inport
  platform_dxdy_cntr_param : Inport  Port=2
  dvarphi_sp : Inport  Port=3
  ena_w : Inport  Port=4
  dvarphi : Inport  Port=5
  Sum : Sum  Inputs=-+|
  Wheels Velocity controller : Subsystem
  varphi_tau_setp_out : Outport
  wires:
  Wheels Velocity controller/1(varphi_tau_setp) -> varphi_tau_setp_out/1
  ena_w/1 -> Wheels Velocity controller/2(ena_w)
  Sum/1 -> Wheels Velocity controller/1(dvarphi_error)
  dvarphi/1 -> Sum/1
  dvarphi_sp/1 -> Sum/2
  disable/1 -> Wheels Velocity controller/4(reset_int)
  platform_dxdy_cntr_param/1 -> Wheels Velocity controller/3(platform_dvarphi_cntr_param)

== system ROPOD_4Wheel_TdistZMPC_cntr_EC/Non-ROS Ropod Controller/ROPOD 4SW TORQUE_MODE/Initialization switch ==
  vel_mode_enable : Inport
  In2 : Inport  Port=2
  Constant13 : Constant  Value=SW_COM1_MODE_TORQUE
  Constant5 : Constant  Value=SW_COM1_MODE_VELOCITY
  Movinf around SW axis center : Constant  Value=[2 -2 2 -2 2 -2 2 -2]
  Switch : Switch  Criteria=u2 ~= 0
  Switch1 : Switch  Criteria=u2 ~= 0
  cntr_mode : Outport
  wheel_setp : Outport  Port=2
  wires:
  Constant13/1 -> Switch/3
  Constant5/1 -> Switch/1
  vel_mode_enable/1 -> Switch/2, Switch1/2
  Switch1/1 -> wheel_setp/1
  Switch/1 -> cntr_mode/1
  Movinf around SW axis center/1 -> Switch1/1
  In2/1 -> Switch1/3

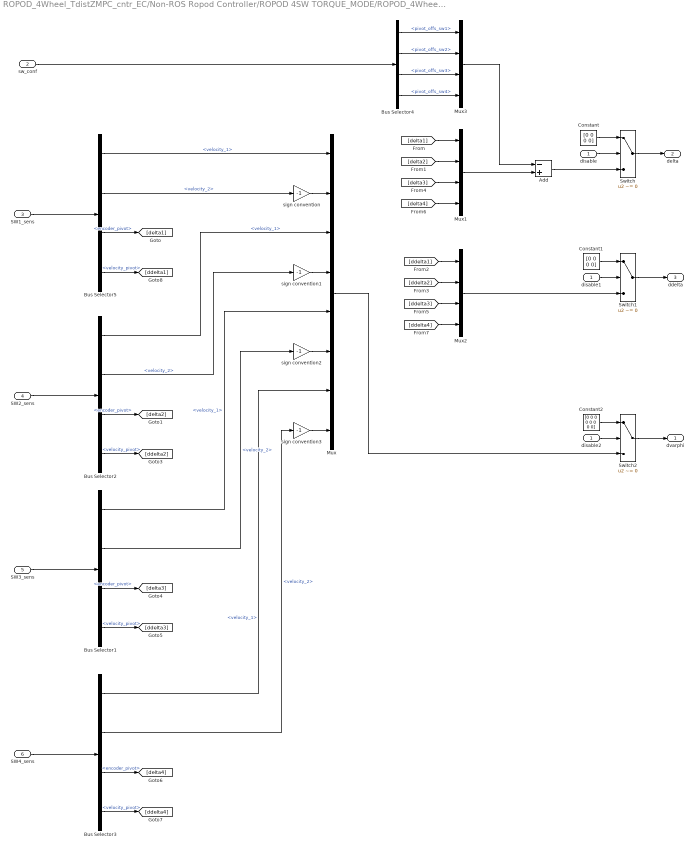
== system ROPOD_4Wheel_TdistZMPC_cntr_EC/Non-ROS Ropod Controller/ROPOD 4SW TORQUE_MODE/ROPOD_4Wheel_sens ==
  disable : Inport
  sw_conf : Inport  Port=2
  SW1_sens : Inport  Port=3
  SW2_sens : Inport  Port=4
  SW3_sens : Inport  Port=5
  SW4_sens : Inport  Port=6
  Add : Sum  Inputs=-+
  Bus Selector{1..3,5} (4 alike) : BusSelector  OutputSignals=velocity_1,velocity_2,encoder_pivot,velocity_pivot
  Bus Selector4 : BusSelector  OutputSignals=pivot_offs_sw1,pivot_offs_sw2,pivot_offs_sw3,pivot_offs_sw4
  Constant : Constant  Value=[0 0 0 0]
  Constant1 : Constant  Value=[0 0 0 0]
  Constant2 : Constant  Value=[0 0 0 0 0 0 0 0]
  Mux : Mux  Inputs=8
  Mux1 : Mux
  Mux2 : Mux
  Mux3 : Mux
  Switch : Switch  Criteria=u2 ~= 0
  Switch1 : Switch  Criteria=u2 ~= 0
  Switch2 : Switch  Criteria=u2 ~= 0
  disable1 : InportShadow
  disable2 : InportShadow
  sign convention{,1..3} (4 alike) : Gain  Gain=-1
  dvarphi : Outport
  delta : Outport  Port=2
  ddelta : Outport  Port=3
  wires:
  SW1_sens/1 -> Bus Selector5/1
  SW2_sens/1 -> Bus Selector2/1
  Bus Selector5/1 -> Mux/1  "<velocity_1>"
  Bus Selector5/2 -> sign convention/1  "<velocity_2>"
  Bus Selector2/1 -> Mux/3  "<velocity_1>"
  Bus Selector2/2 -> sign convention1/1  "<velocity_2>"
  Bus Selector2/3 -> [delta2]  "<encoder_pivot>"
  [delta1] -> Mux1/1
  [delta2] -> Mux1/2
  Bus Selector2/4 -> [ddelta2]  "<velocity_pivot>"
  [ddelta2] -> Mux2/2
  [ddelta1] -> Mux2/1
  Bus Selector1/4 -> [ddelta3]  "<velocity_pivot>"
  Bus Selector1/3 -> [delta3]  "<encoder_pivot>"
  Bus Selector1/2 -> sign convention2/1  "<velocity_2>"
  Bus Selector1/1 -> Mux/5  "<velocity_1>"
  SW3_sens/1 -> Bus Selector1/1
  [delta3] -> Mux1/3
  [ddelta3] -> Mux2/3
  SW4_sens/1 -> Bus Selector3/1
  Bus Selector3/1 -> Mux/7  "<velocity_1>"
  Bus Selector3/2 -> sign convention3/1  "<velocity_2>"
  Bus Selector3/3 -> [delta4]  "<encoder_pivot>"
  Bus Selector3/4 -> [ddelta4]  "<velocity_pivot>"
  [delta4] -> Mux1/4
  [ddelta4] -> Mux2/4
  Mux1/1 -> Add/2
  Mux3/1 -> Add/1
  sw_conf/1 -> Bus Selector4/1
  Bus Selector4/1 -> Mux3/1  "<pivot_offs_sw1>"
  Bus Selector4/2 -> Mux3/2  "<pivot_offs_sw2>"
  Bus Selector4/3 -> Mux3/3  "<pivot_offs_sw3>"
  Bus Selector4/4 -> Mux3/4  "<pivot_offs_sw4>"
  Bus Selector5/3 -> [delta1]  "<encoder_pivot>"
  Bus Selector5/4 -> [ddelta1]  "<velocity_pivot>"
  sign convention/1 -> Mux/2
  sign convention1/1 -> Mux/4
  sign convention2/1 -> Mux/6
  sign convention3/1 -> Mux/8
  Add/1 -> Switch/3
  Switch/1 -> delta/1
  disable/1 -> Switch/2
  Constant/1 -> Switch/1
  Switch1/1 -> ddelta/1
  Mux2/1 -> Switch1/3
  Constant1/1 -> Switch1/1
  disable1/1 -> Switch1/2
  disable2/1 -> Switch2/2
  Constant2/1 -> Switch2/1
  Mux/1 -> Switch2/3
  Switch2/1 -> dvarphi/1

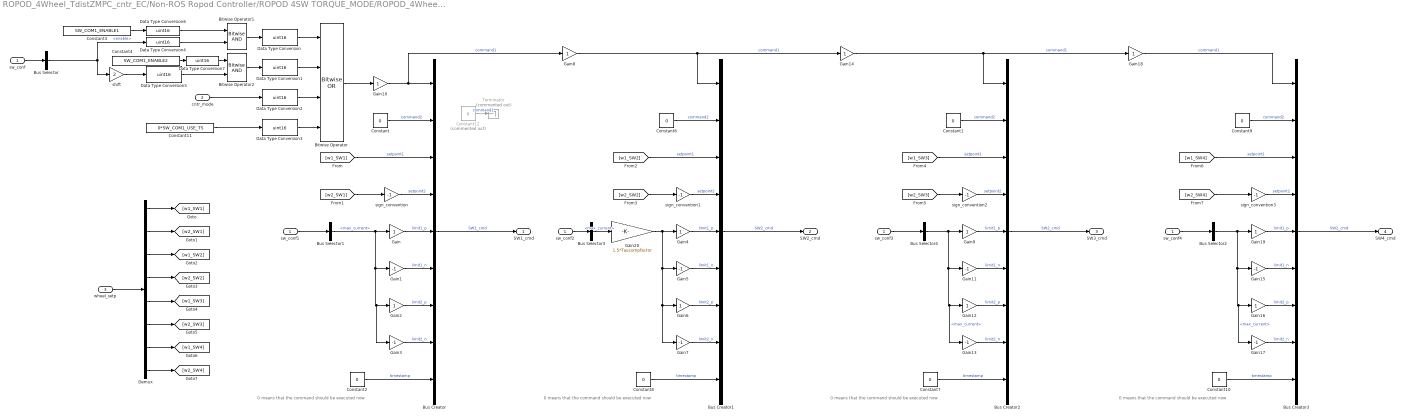
== system ROPOD_4Wheel_TdistZMPC_cntr_EC/Non-ROS Ropod Controller/ROPOD 4SW TORQUE_MODE/ROPOD_4Wheel_torque_cmd ==
  note: 0 means that the command should be executed now
  note: 0 means that the command should be executed now
  note: 0 means that the command should be executed now
  note: 0 means that the command should be executed now
  sw_conf : Inport
  cntr_mode : Inport  Port=2
  wheel_setp : Inport  Port=3
  Bitwise Operator : simulink/Logic and Bit Operations/Bitwise Operator  logicop=OR  UseBitMask=off  NumInputPorts=4  BitMask=bin2dec('11011001')  BitMaskRealWorld=Stored Integer
  Bitwise Operator1 : simulink/Logic and Bit Operations/Bitwise Operator  logicop=AND  UseBitMask=off  NumInputPorts=2  BitMask=bin2dec('11011001')  BitMaskRealWorld=Stored Integer
  Bitwise Operator2 : simulink/Logic and Bit Operations/Bitwise Operator  logicop=AND  UseBitMask=off  NumInputPorts=2  BitMask=bin2dec('11011001')  BitMaskRealWorld=Stored Integer
  Bus Creator{,1..3} (4 alike) : BusCreator  Inputs=9
  Bus Selector : BusSelector  OutputSignals=enable
  Bus Selector{1..4} (4 alike) : BusSelector  OutputSignals=max_current
  Constant{,1..2,6..10} (8 alike) : Constant  Value=0
  Constant11 : Constant  Value=0*SW_COM1_USE_TS
  Constant12 : Constant  Commented=on  Value=8
  Constant3 : Constant  Value=SW_COM1_ENABLE1
  Constant4 : Constant  Value=SW_COM1_ENABLE2
  Data Type Conversion{,1..7} (8 alike) : DataTypeConversion  OutDataTypeStr=uint16
  Demux : Demux  Outputs=8
  Gain{,2,4,6,9,12,16,19} (8 alike) : Gain
  Gain{1,3,5,7,11,13,15,17} (8 alike) : Gain  Gain=-1
  Gain{8,10,14,18} (4 alike) : Gain  OutDataTypeStr=double
  Gain20 : Gain  Gain=1.5*Taucompfactor
  Terminator : Terminator  Commented=on
  shift : Gain  Gain=2
  sign_convention{,1..3} (4 alike) : Gain  Gain=-1
  sw_conf{1..4} (4 alike) : InportShadow
  SW1_cmd : Outport
  SW2_cmd : Outport  Port=2
  SW3_cmd : Outport  Port=3
  SW4_cmd : Outport  Port=4
  wires:
  Bus Creator/1 -> SW1_cmd/1  "SW1_cmd"
  Constant2/1 -> Bus Creator/9  "timestamp"
  Constant/1 -> Bus Creator/2  "command2"
  [w1_SW1] -> Bus Creator/3  "setpoint1"
  Bus Selector1/1 -> Gain3/1, Gain2/1, Gain1/1, Gain/1  "<max_current>"
  [w2_SW1] -> sign_convention/1
  [w2_SW2] -> sign_convention1/1
  [w1_SW2] -> Bus Creator1/3  "setpoint1"
  Constant6/1 -> Bus Creator1/2  "command2"
  Constant8/1 -> Bus Creator1/9  "timestamp"
  Bus Creator1/1 -> SW2_cmd/1  "SW2_cmd"
  Demux/4 -> [w2_SW2]
  Demux/1 -> [w1_SW1]
  Demux/2 -> [w2_SW1]
  Demux/3 -> [w1_SW2]
  wheel_setp/1 -> Demux/1
  Gain/1 -> Bus Creator/5  "limit1_p"
  Gain1/1 -> Bus Creator/6  "limit1_n"
  Gain2/1 -> Bus Creator/7  "limit2_p"
  Gain3/1 -> Bus Creator/8  "limit2_n"
  Gain6/1 -> Bus Creator1/7  "limit2_p"
  Gain4/1 -> Bus Creator1/5  "limit1_p"
  Gain5/1 -> Bus Creator1/6  "limit1_n"
  Gain7/1 -> Bus Creator1/8  "limit2_n"
  Bus Selector3/1 -> Gain20/1  "<max_current>"
  Gain8/1 -> Gain14/1, Bus Creator1/1  "command1"
  Bitwise Operator/1 -> Gain10/1
  Bitwise Operator1/1 -> Data Type Conversion/1
  Data Type Conversion2/1 -> Bitwise Operator/3
  Data Type Conversion1/1 -> Bitwise Operator/2
  Data Type Conversion3/1 -> Bitwise Operator/4
  Bitwise Operator2/1 -> Data Type Conversion1/1
  Data Type Conversion/1 -> Bitwise Operator/1
  Constant11/1 -> Data Type Conversion3/1
  sw_conf/1 -> Bus Selector/1
  Bus Selector/1 -> Data Type Conversion4/1, shift/1  "<enable>"
  sw_conf1/1 -> Bus Selector1/1
  Gain10/1 -> Bus Creator/1, Gain8/1  "command1"
  sw_conf2/1 -> Bus Selector3/1
  Gain12/1 -> Bus Creator2/7  "limit2_p"
  [w2_SW3] -> sign_convention2/1
  Bus Creator2/1 -> SW3_cmd/1  "SW2_cmd"
  Gain13/1 -> Bus Creator2/8  "limit2_n"
  sw_conf3/1 -> Bus Selector4/1
  Gain11/1 -> Bus Creator2/6  "limit1_n"
  Constant1/1 -> Bus Creator2/2  "command2"
  [w1_SW3] -> Bus Creator2/3  "setpoint1"
  Constant7/1 -> Bus Creator2/9  "timestamp"
  Bus Selector4/1 -> Gain13/1, Gain12/1, Gain11/1, Gain9/1  "<max_current>"
  Gain9/1 -> Bus Creator2/5  "limit1_p"
  Demux/5 -> [w1_SW3]
  Demux/6 -> [w2_SW3]
  Gain19/1 -> Bus Creator3/5  "limit1_p"
  Bus Selector2/1 -> Gain19/1, Gain15/1, Gain16/1, Gain17/1  "<max_current>"
  Constant10/1 -> Bus Creator3/9  "timestamp"
  [w1_SW4] -> Bus Creator3/3  "setpoint1"
  Constant9/1 -> Bus Creator3/2  "command2"
  Gain15/1 -> Bus Creator3/6  "limit1_n"
  sw_conf4/1 -> Bus Selector2/1
  Gain17/1 -> Bus Creator3/8  "limit2_n"
  Bus Creator3/1 -> SW4_cmd/1  "SW2_cmd"
  [w2_SW4] -> sign_convention3/1
  Gain16/1 -> Bus Creator3/7  "limit2_p"
  Gain18/1 -> Bus Creator3/1  "command1"
  Gain14/1 -> Gain18/1, Bus Creator2/1  "command1"
  Demux/7 -> [w1_SW4]
  Demux/8 -> [w2_SW4]
  shift/1 -> Data Type Conversion5/1
  Data Type Conversion4/1 -> Bitwise Operator1/2
  Data Type Conversion5/1 -> Bitwise Operator2/2
  Constant3/1 -> Data Type Conversion6/1
  Data Type Conversion6/1 -> Bitwise Operator1/1
  Constant4/1 -> Data Type Conversion7/1
  Data Type Conversion7/1 -> Bitwise Operator2/1
  sign_convention/1 -> Bus Creator/4  "setpoint2"
  sign_convention1/1 -> Bus Creator1/4  "setpoint2"
  sign_convention2/1 -> Bus Creator2/4  "setpoint2"
  sign_convention3/1 -> Bus Creator3/4  "setpoint2"
  Constant12/1 -> Terminator/1  "command1"
  cntr_mode/1 -> Data Type Conversion2/1
  Gain20/1 -> Gain7/1, Gain6/1, Gain5/1, Gain4/1

== system ROPOD_4Wheel_TdistZMPC_cntr_EC/Non-ROS Ropod Controller/ROPOD 4SW TORQUE_MODE/Smart_Wheel_1 ==
  SW1_cmd : Inport
  Bus Creator1 : BusCreator  Inputs=40
  Bus Selector : BusSelector  OutputSignals=command1,command2,setpoint1,setpoint2,limit1_p,limit1_n,limit2_p,limit2_n,timestamp
  ec_ROPOD_SmartWheel : SOEM_EtherCAT_Lib/ec_ROPOD_SmartWheel  link_id=1
      settings: SourceProductName=SOEM_EtherCAT_Lib
  SW1_sens : Outport
  wires:
  Bus Creator1/1 -> SW1_sens/1
  ec_ROPOD_SmartWheel/21 -> Bus Creator1/21  "current_2_u"
  ec_ROPOD_SmartWheel/3 -> Bus Creator1/3  "sensor_ts"
  ec_ROPOD_SmartWheel/34 -> Bus Creator1/34  "accel_y"
  ec_ROPOD_SmartWheel/29 -> Bus Creator1/29  "encoder_pivot"
  ec_ROPOD_SmartWheel/18 -> Bus Creator1/18  "velocity_2"
  ec_ROPOD_SmartWheel/19 -> Bus Creator1/19  "current_2_d"
  ec_ROPOD_SmartWheel/14 -> Bus Creator1/14  "voltage_1_v"
  ec_ROPOD_SmartWheel/6 -> Bus Creator1/6  "velocity_1"
  ec_ROPOD_SmartWheel/12 -> Bus Creator1/12  "voltage_1"
  ec_ROPOD_SmartWheel/35 -> Bus Creator1/35  "accel_z"
  ec_ROPOD_SmartWheel/2 -> Bus Creator1/2  "status2"
  ec_ROPOD_SmartWheel/1 -> Bus Creator1/1  "status1"
  ec_ROPOD_SmartWheel/22 -> Bus Creator1/22  "current_2_v"
  ec_ROPOD_SmartWheel/25 -> Bus Creator1/25  "voltage_2_u"
  ec_ROPOD_SmartWheel/24 -> Bus Creator1/24  "voltage_2"
  ec_ROPOD_SmartWheel/15 -> Bus Creator1/15  "voltage_1_w"
  ec_ROPOD_SmartWheel/9 -> Bus Creator1/9  "current_1_u"
  ec_ROPOD_SmartWheel/28 -> Bus Creator1/28  "temperature_2"
  ec_ROPOD_SmartWheel/37 -> Bus Creator1/37  "gyro_y"
  ec_ROPOD_SmartWheel/20 -> Bus Creator1/20  "current_2_q"
  ec_ROPOD_SmartWheel/38 -> Bus Creator1/38  "gyro_z"
  ec_ROPOD_SmartWheel/13 -> Bus Creator1/13  "voltage_1_u"
  ec_ROPOD_SmartWheel/27 -> Bus Creator1/27  "voltage_2_w"
  ec_ROPOD_SmartWheel/7 -> Bus Creator1/7  "current_1_d"
  ec_ROPOD_SmartWheel/5 -> Bus Creator1/5  "encoder_1"
  ec_ROPOD_SmartWheel/36 -> Bus Creator1/36  "gyro_x"
  ec_ROPOD_SmartWheel/23 -> Bus Creator1/23  "current_2_w"
  ec_ROPOD_SmartWheel/4 -> Bus Creator1/4  "setpoint_ts"
  ec_ROPOD_SmartWheel/17 -> Bus Creator1/17  "encoder_2"
  ec_ROPOD_SmartWheel/11 -> Bus Creator1/11  "current_1_w"
  ec_ROPOD_SmartWheel/40 -> Bus Creator1/40  "pressure"
  ec_ROPOD_SmartWheel/30 -> Bus Creator1/30  "velocity_pivot"
  ec_ROPOD_SmartWheel/10 -> Bus Creator1/10  "current_1_v"
  ec_ROPOD_SmartWheel/39 -> Bus Creator1/39  "temperature_imu"
  ec_ROPOD_SmartWheel/16 -> Bus Creator1/16  "temperature_1"
  ec_ROPOD_SmartWheel/33 -> Bus Creator1/33  "accel_x"
  ec_ROPOD_SmartWheel/26 -> Bus Creator1/26  "voltage_2_v"
  ec_ROPOD_SmartWheel/8 -> Bus Creator1/8  "current_1_q"
  ec_ROPOD_SmartWheel/31 -> Bus Creator1/31  "voltage_bus"
  ec_ROPOD_SmartWheel/32 -> Bus Creator1/32  "imu_ts"
  SW1_cmd/1 -> Bus Selector/1
  Bus Selector/1 -> ec_ROPOD_SmartWheel/1  "<command1>"
  Bus Selector/2 -> ec_ROPOD_SmartWheel/2  "<command2>"
  Bus Selector/3 -> ec_ROPOD_SmartWheel/3  "<setpoint1>"
  Bus Selector/4 -> ec_ROPOD_SmartWheel/4  "<setpoint2>"
  Bus Selector/5 -> ec_ROPOD_SmartWheel/5  "<limit1_p>"
  Bus Selector/6 -> ec_ROPOD_SmartWheel/6  "<limit1_n>"
  Bus Selector/7 -> ec_ROPOD_SmartWheel/7  "<limit2_p>"
  Bus Selector/8 -> ec_ROPOD_SmartWheel/8  "<limit2_n>"
  Bus Selector/9 -> ec_ROPOD_SmartWheel/9  "<timestamp>"
